simulink library "uavsimBlockset_UnitVector"  (Simulink 8.0)
settings: Solver=ode45  StartTime=0.0  StopTime=10.0  RelTol=1e-3
libraries: uavsimblockset x1
settings Model: Creator=mstolle  LastModifiedBy=j.bolting

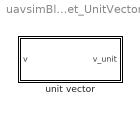
== system uavsimBlockset_UnitVector ==
  unit vector : Subsystem

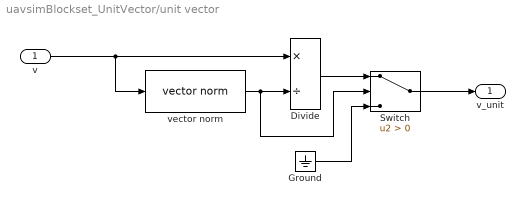
== system uavsimBlockset_UnitVector/unit vector ==
  v : Inport
  Divide : Product  Inputs=*/
  Ground : Ground
  Switch : Switch  Criteria=u2 > Threshold
  vector norm : uavsimblockset/vector norm
  v_unit : Outport
  wires:
  v/1 -> vector norm/1, Divide/1
  vector norm/1 -> Switch/2, Divide/2
  Switch/1 -> v_unit/1
  Divide/1 -> Switch/1
  Ground/1 -> Switch/3
